simulink model "PassengerCar"  (R2019b)
settings: Solver=ode1  StartTime=0  StopTime=25  FixedStep=1.0000000000000000e-003  RelTol=1e-3
InitFcn:
  | sampleTime = str2double(get_param(bdroot, 'FixedStep'));
undefined symbols (not defined in the file or in its folder): AccPedalPos, BrakePedalPos, BrakeSwitch, DiscIntNeverNeededParam, DYNA4, EngSpd, IgnitionSwitch, InitialGear, InitialSpeed, IntendedEngTrq, LeftIndicator, MainBrakePress, MaxGear, MDL, MinGear, RefAcc, RefLane, RefLatPos, RefPath, RefPathCurv, RefSpd, RefSpdPreview, RefSpdRetrospect, RightIndicator, SteeringWheelAng, SteeringWheelTrq, UserDefinedRefValue, vm_const
libraries: UtilitiesLibrary x31, simulink x18, WheelSystemModules x13, LongitudinalControllerModules x13, LateralControllerModules x7, AnimationBusselectorModules x5, EnvironmentModules x5, BasicEngineControlModules x5, MiscellaneousControlModules x5, Animation3Modules x4, AuxiliariesModules x4, TireModules x4
(part 31 of 39)

== system PassengerCar/Vehicle/Drivetrain/DrivetrainPhysics/DrivetrainPhysicsOutputs/Rear3RightShaftOutput ==
  In1 : Inport
  Demux : Demux  Outputs=[1 1 1 1 1]
  Rear3RightShaftOutput : Subsystem  Tag=TESIS DYNAware Interface Block  mask{NeedsUpdate=off, SignalInfo=|}
      mask SignalInfo=|
      | {
      |   "Version": "4.6",
      |   "MuxedOutputBusName": "Rear3RightShaft",
      |   "MuxedInputBusName": "input",
      |   "MuxedInputSelected": false,
      |   "MuxedOutputSelected": true,
      |   "SignalData": [
      |     {
      |       "initialValue": "0.0",
      |       "name": "Trq[Nm]",
      |       "comment": "",
      |       "minString": "",
      |       "maxString": "",
      |       "width": 1,
      |       "dataType": 0,
      |       "signalType": 0,
      |       "createSignal": false,
      |       "outputName": "Trq[Nm]",
      |       "generateSignalAccessBlock": false,
      |       "accessId": "$(parentId).$(blockName).$(outputName)"
      |     },
      |     {
      |       "initialValue": "0.0",
      |       "name": "RotSpdDifferentialOut[rad/s]",
      |       "comment": "",
      |       "minString": "",
      |       "maxString": "",
      |       "width": 1,
      |       "dataType": 0,
      |       "signalType": 0,
      |       "createSignal": false,
      |       "outputName": "RotSpdDifferentialOut[rad/s]",
      |       "generateSignalAccessBlock": false,
      |       "accessId": "$(parentId).$(blockName).$(outputName)"
      |     },
      |     {
      |       "initialValue": "0.0",
      |       "name": "RotAcc[rad/s**2]",
      |       "comment": "",
      |       "minString": "",
      |       "maxString": "",
      |       "width": 1,
      |       "dataType": 0,
      |       "signalType": 0,
      |       "createSignal": false,
      |       "outputName": "RotAcc[rad/s**2]",
      |       "generateSignalAccessBlock": false,
      |       "accessId": "$(parentId).$(blockName).$(outputName)"
      |     },
      |     {
      |       "initialValue": "0.0",
      |       "name": "DerivativeOfTrq_wrt_RotAng[Nm/rad]",
      |       "comment": "",
      |       "minString": "",
      |       "maxString": "",
      |       "width": 1,
      |       "dataType": 0,
      |       "signalType": 0,
      |       "createSignal": false,
      |       "outputName": "DerivativeOfTrq_wrt_RotAng[Nm/rad]",
      |       "generateSignalAccessBlock": false,
      |       "accessId": "$(parentId).$(blockName).$(outputName)"
      |     },
      |     {
      |       "initialValue": "0.0",
      |       "name": "DerivativeOfTrq_wrt_WheelSpd[Nm/(rad/s)]",
      |       "comment": "",
      |       "minString": "",
      |       "maxString": "",
      |       "width": 1,
      |       "dataType": 0,
      |       "signalType": 0,
      |       "createSignal": false,
      |       "outputName": "DerivativeOfTrq_wrt_WheelSpd[Nm/(rad/s)]",
      |       "generateSignalAccessBlock": false,
      |       "accessId": "$(parentId).$(blockName).$(outputName)"
      |     },
      |     {
      |       "initialValue": "0.0",
      |       "name": "AddInrt[kg*m**2]",
      |       "comment": "",
      |       "minString": "",
      |       "maxString": "",
      |       "width": 1,
      |       "dataType": 0,
      |       "signalType": 0,
      |       "createSignal": false,
      |       "outputName": "AddInrt[kg*m**2]",
      |       "generateSignalAccessBlock": false,
      |       "accessId": "$(parentId).$(blockName).$(outputName)"
      |     },
      |     {
      |       "initialValue": "0.0",
      |       "name": "FrictionTrq[Nm]",
      |       "comment": "",
      |       "minString": "",
      |       "maxString": "",
      |       "width": 1,
      |       "dataType": 0,
      |       "signalType": 0,
      |       "createSignal": false,
      |       "outputName": "FrictionTrq[Nm]",
      |       "generateSignalAccessBlock": false,
      |       "accessId": "$(parentId).$(blockName).$(outputName)"
      |     }
      |   ]
      | }
      mask prompts: NeedsUpdate "Specify, if subsystem content needs to be updated"; SignalInfo "Signal Info (json)"
      mask help: DYNA4 Interface Block Version 4.6
      mask init:
      | blockName = get_param(gcbh, 'Name');
      | parentId = DYNA4.ModelHandling.AccessID.getFromHierarchy(gcbh);
      | TD.InterfaceBlock.ModelCallbacks.GenerateContent(gcb);
      settings: DeleteFcn=TD.InterfaceBlock.ModelCallbacks.CloseGUI( gcbh );  NameChangeFcn=TD.InterfaceBlock.ModelCallbacks.BlockRenamedHandler(gcbh);  OpenFcn=TD.InterfaceBlock.ModelCallbacks.OpenGUI( gcbh );  CloseFcn=TD.InterfaceBlock.ModelCallbacks.CloseGUI( gcbh );
      mask Display:
      | image('InterfaceBlock.png','center');
      | port_label('input',1, 'Trq[Nm]');
      | port_label('input',2, 'RotSpdDifferentialOut[rad/s]');
      | port_label('input',3, 'RotAcc[rad/s**2]');
      | port_label('input',4, 'DerivativeOfTrq_wrt_RotAng[Nm/rad]');
      | port_label('input',5, 'DerivativeOfTrq_wrt_WheelSpd[Nm/(rad/s)]');
      | port_label('input',6, 'AddInrt[kg*m**2]');
      | port_label('input',7, 'FrictionTrq[Nm]');
      | port_label('output',1, 'Rear3RightShaft');
  zero : Constant  Value=0
  zero1 : Constant  Value=0
  Rear3RightShaft : Outport  VectorParamsAs1DForOutWhenUnconnected=off
  wires:
  Demux/1 -> Rear3RightShaftOutput/1(Trq[Nm]___UNIQUE_1)
  Demux/2 -> Rear3RightShaftOutput/2(RotSpdDifferentialOut[rad/s]___UNIQUE_1)
  Demux/4 -> Rear3RightShaftOutput/4(DerivativeOfTrq_wrt_RotAng[Nm/rad]___UNIQUE_1)
  Demux/5 -> Rear3RightShaftOutput/5(DerivativeOfTrq_wrt_WheelSpd[Nm/(rad/s)]___UNIQUE_1)
  zero/1 -> Rear3RightShaftOutput/6(AddInrt[kg*m**2]___UNIQUE_1)
  zero1/1 -> Rear3RightShaftOutput/7(FrictionTrq[Nm]___UNIQUE_1)
  Demux/3 -> Rear3RightShaftOutput/3(RotAcc[rad/s**2]___UNIQUE_1)
  Rear3RightShaftOutput/1(Rear3RightShaft___UNIQUE_1) -> Rear3RightShaft/1
  In1/1 -> Demux/1

== system PassengerCar/Vehicle/Drivetrain/DrivetrainPhysics/DrivetrainPhysicsOutputs/RearDifferentialOutput ==
  In2 : Inport
  RearDifferentialOutput : Subsystem  Tag=TESIS DYNAware Interface Block  mask{NeedsUpdate=off, SignalInfo=|}
      mask SignalInfo=|
      | {
      |   "Version": "4.6",
      |   "MuxedOutputBusName": "RearDifferential",
      |   "MuxedInputBusName": "",
      |   "MuxedInputSelected": false,
      |   "MuxedOutputSelected": true,
      |   "SignalData": [
      |     {
      |       "initialValue": "0.0",
      |       "name": "InSpd[rad/s]",
      |       "comment": "",
      |       "minString": "",
      |       "maxString": "",
      |       "width": 1,
      |       "dataType": 0,
      |       "signalType": 0,
      |       "createSignal": false,
      |       "outputName": "InSpd[rad/s]",
      |       "generateSignalAccessBlock": false,
      |       "accessId": "$(parentId).$(blockName).$(outputName)"
      |     },
      |     {
      |       "initialValue": "0.0",
      |       "name": "LeftOutCutTrq[Nm]",
      |       "comment": "",
      |       "minString": "",
      |       "maxString": "",
      |       "width": 1,
      |       "dataType": 0,
      |       "signalType": 0,
      |       "createSignal": false,
      |       "outputName": "LeftOutCutTrq[Nm]",
      |       "generateSignalAccessBlock": false,
      |       "accessId": "$(parentId).$(blockName).$(outputName)"
      |     },
      |     {
      |       "initialValue": "0.0",
      |       "name": "RightOutCutTrq[Nm]",
      |       "comment": "",
      |       "minString": "",
      |       "maxString": "",
      |       "width": 1,
      |       "dataType": 0,
      |       "signalType": 0,
      |       "createSignal": false,
      |       "outputName": "RightOutCutTrq[Nm]",
      |       "generateSignalAccessBlock": false,
      |       "accessId": "$(parentId).$(blockName).$(outputName)"
      |     },
      |     {
      |       "initialValue": "0.0",
      |       "name": "LossPower[W]",
      |       "comment": "",
      |       "minString": "",
      |       "maxString": "",
      |       "width": 1,
      |       "dataType": 0,
      |       "signalType": 0,
      |       "createSignal": false,
      |       "outputName": "LossPower[W]",
      |       "generateSignalAccessBlock": false,
      |       "accessId": "$(parentId).$(blockName).$(outputName)"
      |     }
      |   ]
      | }
      mask prompts: NeedsUpdate "Specify, if subsystem content needs to be updated"; SignalInfo "Signal Info (json)"
      mask help: DYNA4 Interface Block Version 4.6
      mask init:
      | blockName = get_param(gcbh, 'Name');
      | parentId = DYNA4.ModelHandling.AccessID.getFromHierarchy(gcbh);
      | TD.InterfaceBlock.ModelCallbacks.GenerateContent(gcb);
      settings: DeleteFcn=TD.InterfaceBlock.ModelCallbacks.CloseGUI( gcbh );  NameChangeFcn=TD.InterfaceBlock.ModelCallbacks.BlockRenamedHandler(gcbh);  OpenFcn=TD.InterfaceBlock.ModelCallbacks.OpenGUI( gcbh );  CloseFcn=TD.InterfaceBlock.ModelCallbacks.CloseGUI( gcbh );
      mask Display:
      | image('InterfaceBlock.png','center');
      | port_label('input',1, 'InSpd[rad/s]');
      | port_label('input',2, 'LeftOutCutTrq[Nm]');
      | port_label('input',3, 'RightOutCutTrq[Nm]');
      | port_label('input',4, 'LossPower[W]');
      | port_label('output',1, 'RearDifferential');
  zero : Constant  Value=0
  zero1 : Constant  Value=0
  zero2 : Constant  Value=0
  RearDifferential : Outport  VectorParamsAs1DForOutWhenUnconnected=off
  wires:
  zero1/1 -> RearDifferentialOutput/3(RightOutCutTrq[Nm]___UNIQUE_1)
  zero2/1 -> RearDifferentialOutput/4(LossPower[W]___UNIQUE_1)
  zero/1 -> RearDifferentialOutput/2(LeftOutCutTrq[Nm]___UNIQUE_1)
  RearDifferentialOutput/1(RearDifferential___UNIQUE_1) -> RearDifferential/1
  In2/1 -> RearDifferentialOutput/1(InSpd[rad/s]___UNIQUE_1)

== system PassengerCar/Vehicle/Drivetrain/DrivetrainPhysics/DrivetrainPhysicsOutputs/RearLeftShaftOutput ==
  In1 : Inport
  Demux : Demux  Outputs=[1 1 1 1 1]
  RearLeftShaftOutput : Subsystem  Tag=TESIS DYNAware Interface Block  mask{NeedsUpdate=off, SignalInfo=|}
      mask SignalInfo=|
      | {
      |   "Version": "4.6",
      |   "MuxedOutputBusName": "RearLeftShaft",
      |   "MuxedInputBusName": "input",
      |   "MuxedInputSelected": false,
      |   "MuxedOutputSelected": true,
      |   "SignalData": [
      |     {
      |       "initialValue": "0.0",
      |       "name": "Trq[Nm]",
      |       "comment": "",
      |       "minString": "",
      |       "maxString": "",
      |       "width": 1,
      |       "dataType": 0,
      |       "signalType": 0,
      |       "createSignal": false,
      |       "outputName": "Trq[Nm]",
      |       "generateSignalAccessBlock": false,
      |       "accessId": "$(parentId).$(blockName).$(outputName)"
      |     },
      |     {
      |       "initialValue": "0.0",
      |       "name": "RotSpdDifferentialOut[rad/s]",
      |       "comment": "",
      |       "minString": "",
      |       "maxString": "",
      |       "width": 1,
      |       "dataType": 0,
      |       "signalType": 0,
      |       "createSignal": false,
      |       "outputName": "RotSpdDifferentialOut[rad/s]",
      |       "generateSignalAccessBlock": false,
      |       "accessId": "$(parentId).$(blockName).$(outputName)"
      |     },
      |     {
      |       "initialValue": "0.0",
      |       "name": "RotAcc[rad/s**2]",
      |       "comment": "",
      |       "minString": "",
      |       "maxString": "",
      |       "width": 1,
      |       "dataType": 0,
      |       "signalType": 0,
      |       "createSignal": false,
      |       "outputName": "RotAcc[rad/s**2]",
      |       "generateSignalAccessBlock": false,
      |       "accessId": "$(parentId).$(blockName).$(outputName)"
      |     },
      |     {
      |       "initialValue": "0.0",
      |       "name": "DerivativeOfTrq_wrt_RotAng[Nm/rad]",
      |       "comment": "",
      |       "minString": "",
      |       "maxString": "",
      |       "width": 1,
      |       "dataType": 0,
      |       "signalType": 0,
      |       "createSignal": false,
      |       "outputName": "DerivativeOfTrq_wrt_RotAng[Nm/rad]",
      |       "generateSignalAccessBlock": false,
      |       "accessId": "$(parentId).$(blockName).$(outputName)"
      |     },
      |     {
      |       "initialValue": "0.0",
      |       "name": "DerivativeOfTrq_wrt_WheelSpd[Nm/(rad/s)]",
      |       "comment": "",
      |       "minString": "",
      |       "maxString": "",
      |       "width": 1,
      |       "dataType": 0,
      |       "signalType": 0,
      |       "createSignal": false,
      |       "outputName": "DerivativeOfTrq_wrt_WheelSpd[Nm/(rad/s)]",
      |       "generateSignalAccessBlock": false,
      |       "accessId": "$(parentId).$(blockName).$(outputName)"
      |     },
      |     {
      |       "initialValue": "0.0",
      |       "name": "AddInrt[kg*m**2]",
      |       "comment": "",
      |       "minString": "",
      |       "maxString": "",
      |       "width": 1,
      |       "dataType": 0,
      |       "signalType": 0,
      |       "createSignal": false,
      |       "outputName": "AddInrt[kg*m**2]",
      |       "generateSignalAccessBlock": false,
      |       "accessId": "$(parentId).$(blockName).$(outputName)"
      |     },
      |     {
      |       "initialValue": "0.0",
      |       "name": "FrictionTrq[Nm]",
      |       "comment": "",
      |       "minString": "",
      |       "maxString": "",
      |       "width": 1,
      |       "dataType": 0,
      |       "signalType": 0,
      |       "createSignal": false,
      |       "outputName": "FrictionTrq[Nm]",
      |       "generateSignalAccessBlock": false,
      |       "accessId": "$(parentId).$(blockName).$(outputName)"
      |     }
      |   ]
      | }
      mask prompts: NeedsUpdate "Specify, if subsystem content needs to be updated"; SignalInfo "Signal Info (json)"
      mask help: DYNA4 Interface Block Version 4.6
      mask init:
      | blockName = get_param(gcbh, 'Name');
      | parentId = DYNA4.ModelHandling.AccessID.getFromHierarchy(gcbh);
      | TD.InterfaceBlock.ModelCallbacks.GenerateContent(gcb);
      settings: DeleteFcn=TD.InterfaceBlock.ModelCallbacks.CloseGUI( gcbh );  NameChangeFcn=TD.InterfaceBlock.ModelCallbacks.BlockRenamedHandler(gcbh);  OpenFcn=TD.InterfaceBlock.ModelCallbacks.OpenGUI( gcbh );  CloseFcn=TD.InterfaceBlock.ModelCallbacks.CloseGUI( gcbh );
      mask Display:
      | image('InterfaceBlock.png','center');
      | port_label('input',1, 'Trq[Nm]');
      | port_label('input',2, 'RotSpdDifferentialOut[rad/s]');
      | port_label('input',3, 'RotAcc[rad/s**2]');
      | port_label('input',4, 'DerivativeOfTrq_wrt_RotAng[Nm/rad]');
      | port_label('input',5, 'DerivativeOfTrq_wrt_WheelSpd[Nm/(rad/s)]');
      | port_label('input',6, 'AddInrt[kg*m**2]');
      | port_label('input',7, 'FrictionTrq[Nm]');
      | port_label('output',1, 'RearLeftShaft');
  zero : Constant  Value=0
  zero1 : Constant  Value=0
  RearLeftShaft : Outport  VectorParamsAs1DForOutWhenUnconnected=off
  wires:
  In1/1 -> Demux/1
  RearLeftShaftOutput/1(RearLeftShaft___UNIQUE_1) -> RearLeftShaft/1
  Demux/3 -> RearLeftShaftOutput/3(RotAcc[rad/s**2]___UNIQUE_1)
  zero1/1 -> RearLeftShaftOutput/7(FrictionTrq[Nm]___UNIQUE_1)
  zero/1 -> RearLeftShaftOutput/6(AddInrt[kg*m**2]___UNIQUE_1)
  Demux/5 -> RearLeftShaftOutput/5(DerivativeOfTrq_wrt_WheelSpd[Nm/(rad/s)]___UNIQUE_1)
  Demux/4 -> RearLeftShaftOutput/4(DerivativeOfTrq_wrt_RotAng[Nm/rad]___UNIQUE_1)
  Demux/2 -> RearLeftShaftOutput/2(RotSpdDifferentialOut[rad/s]___UNIQUE_1)
  Demux/1 -> RearLeftShaftOutput/1(Trq[Nm]___UNIQUE_1)

== system PassengerCar/Vehicle/Drivetrain/DrivetrainPhysics/DrivetrainPhysicsOutputs/RearRightShaftOutput ==
  In1 : Inport
  Demux : Demux  Outputs=[1 1 1 1 1]
  RearRightShaftOutput : Subsystem  Tag=TESIS DYNAware Interface Block  mask{NeedsUpdate=off, SignalInfo=|}
      mask SignalInfo=|
      | {
      |   "Version": "4.6",
      |   "MuxedOutputBusName": "RearRightShaft",
      |   "MuxedInputBusName": "input",
      |   "MuxedInputSelected": false,
      |   "MuxedOutputSelected": true,
      |   "SignalData": [
      |     {
      |       "initialValue": "0.0",
      |       "name": "Trq[Nm]",
      |       "comment": "",
      |       "minString": "",
      |       "maxString": "",
      |       "width": 1,
      |       "dataType": 0,
      |       "signalType": 0,
      |       "createSignal": false,
      |       "outputName": "Trq[Nm]",
      |       "generateSignalAccessBlock": false,
      |       "accessId": "$(parentId).$(blockName).$(outputName)"
      |     },
      |     {
      |       "initialValue": "0.0",
      |       "name": "RotSpdDifferentialOut[rad/s]",
      |       "comment": "",
      |       "minString": "",
      |       "maxString": "",
      |       "width": 1,
      |       "dataType": 0,
      |       "signalType": 0,
      |       "createSignal": false,
      |       "outputName": "RotSpdDifferentialOut[rad/s]",
      |       "generateSignalAccessBlock": false,
      |       "accessId": "$(parentId).$(blockName).$(outputName)"
      |     },
      |     {
      |       "initialValue": "0.0",
      |       "name": "RotAcc[rad/s**2]",
      |       "comment": "",
      |       "minString": "",
      |       "maxString": "",
      |       "width": 1,
      |       "dataType": 0,
      |       "signalType": 0,
      |       "createSignal": false,
      |       "outputName": "RotAcc[rad/s**2]",
      |       "generateSignalAccessBlock": false,
      |       "accessId": "$(parentId).$(blockName).$(outputName)"
      |     },
      |     {
      |       "initialValue": "0.0",
      |       "name": "DerivativeOfTrq_wrt_RotAng[Nm/rad]",
      |       "comment": "",
      |       "minString": "",
      |       "maxString": "",
      |       "width": 1,
      |       "dataType": 0,
      |       "signalType": 0,
      |       "createSignal": false,
      |       "outputName": "DerivativeOfTrq_wrt_RotAng[Nm/rad]",
      |       "generateSignalAccessBlock": false,
      |       "accessId": "$(parentId).$(blockName).$(outputName)"
      |     },
      |     {
      |       "initialValue": "0.0",
      |       "name": "DerivativeOfTrq_wrt_WheelSpd[Nm/(rad/s)]",
      |       "comment": "",
      |       "minString": "",
      |       "maxString": "",
      |       "width": 1,
      |       "dataType": 0,
      |       "signalType": 0,
      |       "createSignal": false,
      |       "outputName": "DerivativeOfTrq_wrt_WheelSpd[Nm/(rad/s)]",
      |       "generateSignalAccessBlock": false,
      |       "accessId": "$(parentId).$(blockName).$(outputName)"
      |     },
      |     {
      |       "initialValue": "0.0",
      |       "name": "AddInrt[kg*m**2]",
      |       "comment": "",
      |       "minString": "",
      |       "maxString": "",
      |       "width": 1,
      |       "dataType": 0,
      |       "signalType": 0,
      |       "createSignal": false,
      |       "outputName": "AddInrt[kg*m**2]",
      |       "generateSignalAccessBlock": false,
      |       "accessId": "$(parentId).$(blockName).$(outputName)"
      |     },
      |     {
      |       "initialValue": "0.0",
      |       "name": "FrictionTrq[Nm]",
      |       "comment": "",
      |       "minString": "",
      |       "maxString": "",
      |       "width": 1,
      |       "dataType": 0,
      |       "signalType": 0,
      |       "createSignal": false,
      |       "outputName": "FrictionTrq[Nm]",
      |       "generateSignalAccessBlock": false,
      |       "accessId": "$(parentId).$(blockName).$(outputName)"
      |     }
      |   ]
      | }
      mask prompts: NeedsUpdate "Specify, if subsystem content needs to be updated"; SignalInfo "Signal Info (json)"
      mask help: DYNA4 Interface Block Version 4.6
      mask init:
      | blockName = get_param(gcbh, 'Name');
      | parentId = DYNA4.ModelHandling.AccessID.getFromHierarchy(gcbh);
      | TD.InterfaceBlock.ModelCallbacks.GenerateContent(gcb);
      settings: DeleteFcn=TD.InterfaceBlock.ModelCallbacks.CloseGUI( gcbh );  NameChangeFcn=TD.InterfaceBlock.ModelCallbacks.BlockRenamedHandler(gcbh);  OpenFcn=TD.InterfaceBlock.ModelCallbacks.OpenGUI( gcbh );  CloseFcn=TD.InterfaceBlock.ModelCallbacks.CloseGUI( gcbh );
      mask Display:
      | image('InterfaceBlock.png','center');
      | port_label('input',1, 'Trq[Nm]');
      | port_label('input',2, 'RotSpdDifferentialOut[rad/s]');
      | port_label('input',3, 'RotAcc[rad/s**2]');
      | port_label('input',4, 'DerivativeOfTrq_wrt_RotAng[Nm/rad]');
      | port_label('input',5, 'DerivativeOfTrq_wrt_WheelSpd[Nm/(rad/s)]');
      | port_label('input',6, 'AddInrt[kg*m**2]');
      | port_label('input',7, 'FrictionTrq[Nm]');
      | port_label('output',1, 'RearRightShaft');
  zero : Constant  Value=0
  zero1 : Constant  Value=0
  RearRightShaft : Outport  VectorParamsAs1DForOutWhenUnconnected=off
  wires:
  Demux/1 -> RearRightShaftOutput/1(Trq[Nm]___UNIQUE_1)
  Demux/2 -> RearRightShaftOutput/2(RotSpdDifferentialOut[rad/s]___UNIQUE_1)
  Demux/4 -> RearRightShaftOutput/4(DerivativeOfTrq_wrt_RotAng[Nm/rad]___UNIQUE_1)
  Demux/5 -> RearRightShaftOutput/5(DerivativeOfTrq_wrt_WheelSpd[Nm/(rad/s)]___UNIQUE_1)
  zero/1 -> RearRightShaftOutput/6(AddInrt[kg*m**2]___UNIQUE_1)
  zero1/1 -> RearRightShaftOutput/7(FrictionTrq[Nm]___UNIQUE_1)
  Demux/3 -> RearRightShaftOutput/3(RotAcc[rad/s**2]___UNIQUE_1)
  RearRightShaftOutput/1(RearRightShaft___UNIQUE_1) -> RearRightShaft/1
  In1/1 -> Demux/1

== system PassengerCar/Vehicle/Drivetrain/DrivetrainPhysics/DrivetrainPhysicsOutputs/TransferCaseOutput ==
  In2 : Inport
  TransferCaseOutput : Subsystem  Tag=TESIS DYNAware Interface Block  mask{NeedsUpdate=off, SignalInfo=|}
      mask SignalInfo=|
      | {
      |   "Version": "4.6",
      |   "MuxedOutputBusName": "TransferCase",
      |   "MuxedInputBusName": "input",
      |   "MuxedInputSelected": false,
      |   "MuxedOutputSelected": true,
      |   "SignalData": [
      |     {
      |       "initialValue": "0.0",
      |       "name": "InSpd[rad/s]",
      |       "comment": "",
      |       "minString": "",
      |       "maxString": "",
      |       "width": 1,
      |       "dataType": 0,
      |       "signalType": 0,
      |       "createSignal": false,
      |       "outputName": "InSpd[rad/s]",
      |       "generateSignalAccessBlock": false,
      |       "accessId": "$(parentId).$(blockName).$(outputName)"
      |     },
      |     {
      |       "initialValue": "0.0",
      |       "name": "FrontOutCutTrq[Nm]",
      |       "comment": "",
      |       "minString": "",
      |       "maxString": "",
      |       "width": 1,
      |       "dataType": 0,
      |       "signalType": 0,
      |       "createSignal": false,
      |       "outputName": "FrontOutCutTrq[Nm]",
      |       "generateSignalAccessBlock": false,
      |       "accessId": "$(parentId).$(blockName).$(outputName)"
      |     },
      |     {
      |       "initialValue": "0.0",
      |       "name": "RearOutCutTrq[Nm]",
      |       "comment": "",
      |       "minString": "",
      |       "maxString": "",
      |       "width": 1,
      |       "dataType": 0,
      |       "signalType": 0,
      |       "createSignal": false,
      |       "outputName": "RearOutCutTrq[Nm]",
      |       "generateSignalAccessBlock": false,
      |       "accessId": "$(parentId).$(blockName).$(outputName)"
      |     },
      |     {
      |       "initialValue": "0.0",
      |       "name": "LossPower[W]",
      |       "comment": "",
      |       "minString": "",
      |       "maxString": "",
      |       "width": 1,
      |       "dataType": 0,
      |       "signalType": 0,
      |       "createSignal": false,
      |       "outputName": "LossPower[W]",
      |       "generateSignalAccessBlock": false,
      |       "accessId": "$(parentId).$(blockName).$(outputName)"
      |     }
      |   ]
      | }
      mask prompts: NeedsUpdate "Specify, if subsystem content needs to be updated"; SignalInfo "Signal Info (json)"
      mask help: DYNA4 Interface Block Version 4.6
      mask init:
      | blockName = get_param(gcbh, 'Name');
      | parentId = DYNA4.ModelHandling.AccessID.getFromHierarchy(gcbh);
      | TD.InterfaceBlock.ModelCallbacks.GenerateContent(gcb);
      settings: DeleteFcn=TD.InterfaceBlock.ModelCallbacks.CloseGUI( gcbh );  NameChangeFcn=TD.InterfaceBlock.ModelCallbacks.BlockRenamedHandler(gcbh);  OpenFcn=TD.InterfaceBlock.ModelCallbacks.OpenGUI( gcbh );  CloseFcn=TD.InterfaceBlock.ModelCallbacks.CloseGUI( gcbh );
      mask Display:
      | image('InterfaceBlock.png','center');
      | port_label('input',1, 'InSpd[rad/s]');
      | port_label('input',2, 'FrontOutCutTrq[Nm]');
      | port_label('input',3, 'RearOutCutTrq[Nm]');
      | port_label('input',4, 'LossPower[W]');
      | port_label('output',1, 'TransferCase');
  zero : Constant  Value=0
  zero1 : Constant  Value=0
  zero2 : Constant  Value=0
  TransferCase : Outport  VectorParamsAs1DForOutWhenUnconnected=off
  wires:
  zero1/1 -> TransferCaseOutput/3(RearOutCutTrq[Nm]___UNIQUE_1)
  zero2/1 -> TransferCaseOutput/4(LossPower[W]___UNIQUE_1)
  zero/1 -> TransferCaseOutput/2(FrontOutCutTrq[Nm]___UNIQUE_1)
  TransferCaseOutput/1(TransferCase___UNIQUE_1) -> TransferCase/1
  In2/1 -> TransferCaseOutput/1(InSpd[rad/s]___UNIQUE_1)

== system PassengerCar/Vehicle/Drivetrain/DrivetrainPhysics/DrivetrainPhysicsOutputs/TransmissionOutput ==
  TransmissionStates : Inport
  Demux : Demux  Outputs=8
  Memory1 : Memory  InheritSampleTime=on
  Memory2 : Memory  InheritSampleTime=on
  Memory3 : Memory  InheritSampleTime=on
  TransmissionOutput : Subsystem  Tag=TESIS DYNAware Interface Block  mask{NeedsUpdate=off, SignalInfo=|}
      mask SignalInfo=|
      | {
      |   "Version": "4.6",
      |   "MuxedOutputBusName": "Transmission",
      |   "MuxedInputBusName": "input",
      |   "MuxedInputSelected": false,
      |   "MuxedOutputSelected": true,
      |   "SignalData": [
      |     {
      |       "initialValue": "0.0",
      |       "name": "NumFwdGears[-]",
      |       "comment": "",
      |       "minString": "",
      |       "maxString": "",
      |       "width": 1,
      |       "dataType": 0,
      |       "signalType": 0,
      |       "createSignal": false,
      |       "outputName": "NumFwdGears[-]",
      |       "generateSignalAccessBlock": false,
      |       "accessId": "$(parentId).$(blockName).$(outputName)"
      |     },
      |     {
      |       "initialValue": "0.0",
      |       "name": "Type[-]",
      |       "comment": "",
      |       "minString": "",
      |       "maxString": "",
      |       "width": 1,
      |       "dataType": 0,
      |       "signalType": 0,
      |       "createSignal": false,
      |       "outputName": "Type[-]",
      |       "generateSignalAccessBlock": false,
      |       "accessId": "$(parentId).$(blockName).$(outputName)"
      |     },
      |     {
      |       "initialValue": "0.0",
      |       "name": "Gear[-4;20]",
      |       "comment": "",
      |       "minString": "",
      |       "maxString": "",
      |       "width": 1,
      |       "dataType": 0,
      |       "signalType": 0,
      |       "createSignal": false,
      |       "outputName": "Gear[-4;20]",
      |       "generateSignalAccessBlock": false,
      |       "accessId": "$(parentId).$(blockName).$(outputName)"
      |     },
      |     {
      |       "initialValue": "0.0",
      |       "name": "InSpd[rad/s]",
      |       "comment": "",
      |       "minString": "",
      |       "maxString": "",
      |       "width": 1,
      |       "dataType": 0,
      |       "signalType": 0,
      |       "createSignal": false,
      |       "outputName": "InSpd[rad/s]",
      |       "generateSignalAccessBlock": false,
      |       "accessId": "$(parentId).$(blockName).$(outputName)"
      |     },
      |     {
      |       "initialValue": "0.0",
      |       "name": "OutSpd[rad/s]",
      |       "comment": "",
      |       "minString": "",
      |       "maxString": "",
      |       "width": 1,
      |       "dataType": 0,
      |       "signalType": 0,
      |       "createSignal": false,
      |       "outputName": "OutSpd[rad/s]",
      |       "generateSignalAccessBlock": false,
      |       "accessId": "$(parentId).$(blockName).$(outputName)"
      |     },
      |     {
      |       "initialValue": "0.0",
      |       "name": "GearChangeTimeConst[s]",
      |       "comment": "",
      |       "minString": "",
      |       "maxString": "",
      |       "width": 1,
      |       "dataType": 0,
      |       "signalType": 0,
      |       "createSignal": false,
      |       "outputName": "GearChangeTimeConst[s]",
      |       "generateSignalAccessBlock": false,
      |       "accessId": "$(parentId).$(blockName).$(outputName)"
      |     },
      |     {
      |       "initialValue": "0.0",
      |       "name": "OutCutTrq[Nm]",
      |       "comment": "",
      |       "minString": "",
      |       "maxString": "",
      |       "width": 1,
      |       "dataType": 0,
      |       "signalType": 0,
      |       "createSignal": false,
      |       "outputName": "OutCutTrq[Nm]",
      |       "generateSignalAccessBlock": false,
      |       "accessId": "$(parentId).$(blockName).$(outputName)"
      |     },
      |     {
      |       "initialValue": "0.0",
      |       "name": "LossPower[W]",
      |       "comment": "",
      |       "minString": "",
      |       "maxString": "",
      |       "width": 1,
      |       "dataType": 0,
      |       "signalType": 0,
      |       "createSignal": false,
      |       "outputName": "LossPower[W]",
      |       "generateSignalAccessBlock": false,
      |       "accessId": "$(parentId).$(blockName).$(outputName)"
      |     },
      |     {
      |       "initialValue": "0.0",
      |       "name": "TurbTrq[Nm]",
      |       "comment": "",
      |       "minString": "",
      |       "maxString": "",
      |       "width": 1,
      |       "dataType": 0,
      |       "signalType": 0,
      |       "createSignal": false,
      |       "outputName": "TurbTrq[Nm]",
      |       "generateSignalAccessBlock": false,
      |       "accessId": "$(parentId).$(blockName).$(outputName)"
      |     },
      |     {
      |       "initialValue": "0.0",
      |       "name": "LockUpClutchPos[0_1]",
      |       "comment": "",
      |       "minString": "",
      |       "maxString": "",
      |       "width": 1,
      |       "dataType": 0,
      |       "signalType": 0,
      |       "createSignal": false,
      |       "outputName": "LockUpClutchPos[0_1]",
      |       "generateSignalAccessBlock": false,
      |       "accessId": "$(parentId).$(blockName).$(outputName)"
      |     }
      |   ]
      | }
      mask prompts: NeedsUpdate "Specify, if subsystem content needs to be updated"; SignalInfo "Signal Info (json)"
      mask help: DYNA4 Interface Block Version 4.6
      mask init:
      | blockName = get_param(gcbh, 'Name');
      | parentId = DYNA4.ModelHandling.AccessID.getFromHierarchy(gcbh);
      | TD.InterfaceBlock.ModelCallbacks.GenerateContent(gcb);
      settings: DeleteFcn=TD.InterfaceBlock.ModelCallbacks.CloseGUI( gcbh );  NameChangeFcn=TD.InterfaceBlock.ModelCallbacks.BlockRenamedHandler(gcbh);  OpenFcn=TD.InterfaceBlock.ModelCallbacks.OpenGUI( gcbh );  CloseFcn=TD.InterfaceBlock.ModelCallbacks.CloseGUI( gcbh );
      mask Display:
      | image('InterfaceBlock.png','center');
      | port_label('input',1, 'NumFwdGears[-]');
      | port_label('input',2, 'Type[-]');
      | port_label('input',3, 'Gear[-4;20]');
      | port_label('input',4, 'InSpd[rad/s]');
      | port_label('input',5, 'OutSpd[rad/s]');
      | port_label('input',6, 'GearChangeTimeConst[s]');
      | port_label('input',7, 'OutCutTrq[Nm]');
      | port_label('input',8, 'LossPower[W]');
      | port_label('input',9, 'TurbTrq[Nm]');
      | port_label('input',10, 'LockUpClutchPos[0_1]');
      | port_label('output',1, 'Transmission');
  zero : Constant  Value=0
  zero1 : Constant  Value=0
  Transmission : Outport  VectorParamsAs1DForOutWhenUnconnected=off
  wires:
  Memory1/1 -> TransmissionOutput/6(GearChangeTimeConst[s]___UNIQUE_1)
  Demux/8 -> Memory1/1
  Demux/5 -> TransmissionOutput/3(Gear[-4;20]___UNIQUE_1)
  Memory2/1 -> TransmissionOutput/5(OutSpd[rad/s]___UNIQUE_1)
  Memory3/1 -> TransmissionOutput/4(InSpd[rad/s]___UNIQUE_1)
  Demux/6 -> Memory3/1
  Demux/7 -> Memory2/1
  Demux/2 -> TransmissionOutput/10(LockUpClutchPos[0_1]___UNIQUE_1)
  Demux/1 -> TransmissionOutput/9(TurbTrq[Nm]___UNIQUE_1)
  TransmissionOutput/1(Transmission___UNIQUE_1) -> Transmission/1
  TransmissionStates/1 -> Demux/1
  Demux/3 -> TransmissionOutput/1(NumFwdGears[-]___UNIQUE_1)
  Demux/4 -> TransmissionOutput/2(Type[-]___UNIQUE_1)
  zero/1 -> TransmissionOutput/7(OutCutTrq[Nm]___UNIQUE_1)
  zero1/1 -> TransmissionOutput/8(LossPower[W]___UNIQUE_1)

== system PassengerCar/Vehicle/WheelSystem/FrontLeftWheelSystem/Tire/DynaComponentInfo ==

== system PassengerCar/Vehicle/WheelSystem/FrontLeftWheelSystem/Tire/InputFromCTRL ==
  fromCTRL : Inport
  TDBusSelector : BusSelector  OutputSignals=AddRoadElev[m],RoadFrictionScaling[0_2],AddLongRoadSlope[-],AddLatRoadSlope[-],LocalRoadSysSwitch[0;1],RelInflPress[Pa]
  __TDD__AddLatRoadSlope[-] : Demux  Outputs=[1]
  __TDD__AddLongRoadSlope[-] : Demux  Outputs=[1]
  __TDD__AddRoadElev[m] : Demux  Outputs=[1]
  __TDD__LocalRoadSysSwitch[0;1] : Demux  Outputs=[1]
  __TDD__RelInflPress[Pa] : Demux  Outputs=1
  __TDD__RoadFrictionScaling[0_2] : Demux  Outputs=[1]
  AddRoadElev[m]___UNIQUE_1 : Outport  Description=|  PortDimensions=[1]  VectorParamsAs1DForOutWhenUnconnected=off
      | <name>AddRoadElev[m]</name>
      | <comment></comment>
  RoadFrictionScaling[0_2]___UNIQUE_1 : Outport  Description=|  Port=2  PortDimensions=[1]  VectorParamsAs1DForOutWhenUnconnected=off
      | <name>RoadFrictionScaling[0_2]</name>
      | <comment></comment>
  AddLongRoadSlope[-]___UNIQUE_1 : Outport  Description=|  Port=3  PortDimensions=[1]  VectorParamsAs1DForOutWhenUnconnected=off
      | <name>AddLongRoadSlope[-]</name>
      | <comment></comment>
  AddLatRoadSlope[-]___UNIQUE_1 : Outport  Description=|  Port=4  PortDimensions=[1]  VectorParamsAs1DForOutWhenUnconnected=off
      | <name>AddLatRoadSlope[-]</name>
      | <comment></comment>
  LocalRoadSysSwitch[0;1]___UNIQUE_1 : Outport  Description=|  Port=5  PortDimensions=[1]  VectorParamsAs1DForOutWhenUnconnected=off
      | <name>LocalRoadSysSwitch[0;1]</name>
      | <comment></comment>
  RelInflPress[Pa]___UNIQUE_1 : Outport  Description=|  Port=6  VectorParamsAs1DForOutWhenUnconnected=off
      | <name>RelInflPress[Pa]</name>
      | <comment></comment>
  wires:
  fromCTRL/1 -> TDBusSelector/1
  TDBusSelector/1 -> __TDD__AddRoadElev[m]/1  "<AddRoadElev[m]>"
  TDBusSelector/2 -> __TDD__RoadFrictionScaling[0_2]/1  "<RoadFrictionScaling[0_2]>"
  TDBusSelector/3 -> __TDD__AddLongRoadSlope[-]/1  "<AddLongRoadSlope[-]>"
  TDBusSelector/4 -> __TDD__AddLatRoadSlope[-]/1  "<AddLatRoadSlope[-]>"
  TDBusSelector/5 -> __TDD__LocalRoadSysSwitch[0;1]/1  "<LocalRoadSysSwitch[0;1]>"
  TDBusSelector/6 -> __TDD__RelInflPress[Pa]/1  "<RelInflPress[Pa]>"
  __TDD__AddRoadElev[m]/1 -> AddRoadElev[m]___UNIQUE_1/1  "AddRoadElev[m]"
  __TDD__RoadFrictionScaling[0_2]/1 -> RoadFrictionScaling[0_2]___UNIQUE_1/1  "RoadFrictionScaling[0_2]"
  __TDD__AddLongRoadSlope[-]/1 -> AddLongRoadSlope[-]___UNIQUE_1/1  "AddLongRoadSlope[-]"
  __TDD__AddLatRoadSlope[-]/1 -> AddLatRoadSlope[-]___UNIQUE_1/1  "AddLatRoadSlope[-]"
  __TDD__LocalRoadSysSwitch[0;1]/1 -> LocalRoadSysSwitch[0;1]___UNIQUE_1/1  "LocalRoadSysSwitch[0;1]"
  __TDD__RelInflPress[Pa]/1 -> RelInflPress[Pa]___UNIQUE_1/1  "RelInflPress[Pa]"

== system PassengerCar/Vehicle/WheelSystem/FrontLeftWheelSystem/Tire/InputFromChassis ==
  fromChassis : Inport
  TDBusSelector : BusSelector  OutputSignals=VehicleBody.Pos(WorldSys)[m],VehicleBody.RotMatrix(WorldSys)[-],WheelSystem.WheelRotAxis(VehSys)[-],WheelSystem.TirePos(VehSys)[m],WheelSystem.TireVel_wrt_WorldSys(VehSys)[m/s],WheelSystem.WheelRotVel_wrt_WorldSys(VehSys)[rad/s]
  __TDD__Pos(WorldSys)[m] : Demux  Outputs=[3]
  __TDD__RotMatrix(WorldSys)[-] : Demux  Outputs=[9]
  __TDD__TirePos(VehSys)[m] : Demux  Outputs=[3]
  __TDD__TireVel_wrt_WorldSys(VehSys)[m/s] : Demux  Outputs=[3]
  __TDD__WheelRotAxis(VehSys)[-] : Demux  Outputs=[3]
  __TDD__WheelRotVel_wrt_WorldSys(VehSys)[rad/s] : Demux  Outputs=[3]
  Pos(WorldSys)[m]___UNIQUE_1 : Outport  Description=|  PortDimensions=[3]  VectorParamsAs1DForOutWhenUnconnected=off
      | <name>VehicleBody.Pos(WorldSys)[m]</name>
      | <comment></comment>
  RotMatrix(WorldSys)[-]___UNIQUE_1 : Outport  Description=|  Port=2  PortDimensions=[9]  VectorParamsAs1DForOutWhenUnconnected=off
      | <name>VehicleBody.RotMatrix(WorldSys)[-]</name>
      | <comment></comment>
  WheelRotAxis(VehSys)[-]___UNIQUE_1 : Outport  Description=|  Port=3  PortDimensions=[3]  VectorParamsAs1DForOutWhenUnconnected=off
      | <name>WheelSystem.WheelRotAxis(VehSys)[-]</name>
      | <comment></comment>
  TirePos(VehSys)[m]___UNIQUE_1 : Outport  Description=|  Port=4  PortDimensions=[3]  VectorParamsAs1DForOutWhenUnconnected=off
      | <name>WheelSystem.TirePos(VehSys)[m]</name>
      | <comment></comment>
  TireVel_wrt_WorldSys(VehSys)[m/s]___UNIQUE_1 : Outport  Description=|  Port=5  PortDimensions=[3]  VectorParamsAs1DForOutWhenUnconnected=off
      | <name>WheelSystem.TireVel_wrt_WorldSys(VehSys)[m/s]</name>
      | <comment></comment>
  WheelRotVel_wrt_WorldSys(VehSys)[rad/s]___UNIQUE_1 : Outport  Description=|  Port=6  PortDimensions=[3]  VectorParamsAs1DForOutWhenUnconnected=off
      | <name>WheelSystem.WheelRotVel_wrt_WorldSys(VehSys)[rad/s]</name>
      | <comment></comment>
  wires:
  fromChassis/1 -> TDBusSelector/1
  TDBusSelector/1 -> __TDD__Pos(WorldSys)[m]/1  "<Pos(WorldSys)[m]>"
  TDBusSelector/2 -> __TDD__RotMatrix(WorldSys)[-]/1  "<RotMatrix(WorldSys)[-]>"
  TDBusSelector/3 -> __TDD__WheelRotAxis(VehSys)[-]/1  "<WheelRotAxis(VehSys)[-]>"
  TDBusSelector/4 -> __TDD__TirePos(VehSys)[m]/1  "<TirePos(VehSys)[m]>"
  TDBusSelector/5 -> __TDD__TireVel_wrt_WorldSys(VehSys)[m/s]/1  "<TireVel_wrt_WorldSys(VehSys)[m/s]>"
  TDBusSelector/6 -> __TDD__WheelRotVel_wrt_WorldSys(VehSys)[rad/s]/1  "<WheelRotVel_wrt_WorldSys(VehSys)[rad/s]>"
  __TDD__Pos(WorldSys)[m]/1 -> Pos(WorldSys)[m]___UNIQUE_1/1  "Pos(WorldSys)[m]"
  __TDD__RotMatrix(WorldSys)[-]/1 -> RotMatrix(WorldSys)[-]___UNIQUE_1/1  "RotMatrix(WorldSys)[-]"
  __TDD__WheelRotAxis(VehSys)[-]/1 -> WheelRotAxis(VehSys)[-]___UNIQUE_1/1  "WheelRotAxis(VehSys)[-]"
  __TDD__TirePos(VehSys)[m]/1 -> TirePos(VehSys)[m]___UNIQUE_1/1  "TirePos(VehSys)[m]"
  __TDD__TireVel_wrt_WorldSys(VehSys)[m/s]/1 -> TireVel_wrt_WorldSys(VehSys)[m/s]___UNIQUE_1/1  "TireVel_wrt_WorldSys(VehSys)[m/s]"
  __TDD__WheelRotVel_wrt_WorldSys(VehSys)[rad/s]/1 -> WheelRotVel_wrt_WorldSys(VehSys)[rad/s]___UNIQUE_1/1  "WheelRotVel_wrt_WorldSys(VehSys)[rad/s]"

== system PassengerCar/Vehicle/WheelSystem/FrontLeftWheelSystem/Tire/InputFromWheel ==
  fromWheel : Inport
  TDBusSelector : BusSelector  OutputSignals=RotSpd[rad/s]
  __TDD__RotSpd[rad/s] : Demux  Outputs=[1]
  RotSpd[rad/s]___UNIQUE_1 : Outport  Description=|  PortDimensions=[1]  VectorParamsAs1DForOutWhenUnconnected=off
      | <name>RotSpd[rad/s]</name>
      | <comment></comment>
  wires:
  fromWheel/1 -> TDBusSelector/1
  TDBusSelector/1 -> __TDD__RotSpd[rad/s]/1  "<RotSpd[rad/s]>"
  __TDD__RotSpd[rad/s]/1 -> RotSpd[rad/s]___UNIQUE_1/1  "RotSpd[rad/s]"
